simulink model "Simulacao"  (R2013b)
settings: Solver=ode45  StartTime=0.0  StopTime=10  RelTol=1e-3
values from neighbouring files (symbols this model uses):
  A = [-1.01887   0.90506   -0.00215 ... (first row only)    [Main.m]
  B = [0  0  20.2]'    [Main.m]
  C = [57.2958      0    0 ... (first row only)    [Main.m]
  D = [0 0]'    [Main.m]
settings Model: Creator=Eduardo  LastModifiedBy=Eduardo

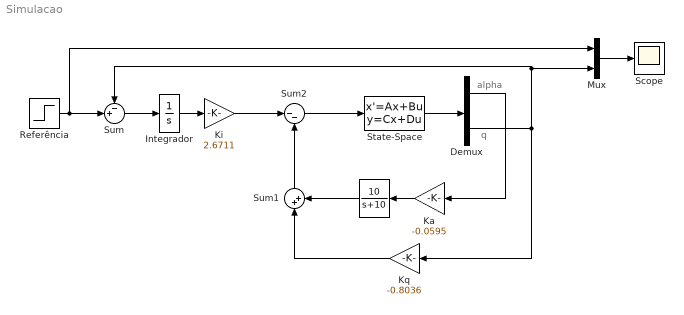
== system Simulacao ==
  note: alpha
  note: q
  " " : TransferFcn  Numerator=[10]  Denominator=[1 10]
  Demux : Demux  Outputs=2
  Integrador : TransferFcn  Denominator=[1 0]
  Ka : Gain  Gain=-0.0595
  Ki : Gain  Gain=2.6711
  Kq : Gain  Gain=-0.8036
  Mux : Mux  Inputs=2
  Referência : Step  SampleTime=0
  Scope : Scope
  State-Space : StateSpace  A=A  B=B  C=C  D=D  X0=0
  Sum : Sum  Inputs=-+|
  Sum1 : Sum  Inputs=|++
  Sum2 : Sum  Inputs=|--
  wires:
  Integrador/1 -> Ki/1
  Ka/1 -> " "/1
  Kq/1 -> Sum1/1
  " "/1 -> Sum1/2
  Ki/1 -> Sum2/1
  Sum1/1 -> Sum2/2
  Referência/1 -> Mux/1, Sum/2
  Sum/1 -> Integrador/1
  Demux/2 -> Kq/1, Sum/1, Mux/2
  Demux/1 -> Ka/1
  Mux/1 -> Scope/1
  Sum2/1 -> State-Space/1
  State-Space/1 -> Demux/1
